simulink model "Systeem_Identificatie_Parameter_Estimation"  (R2018b)
settings: Solver=FixedStepAuto  StartTime=0.0  StopTime=4  FixedStep=1/50000  RelTol=1e-3
values from neighbouring files (symbols this model uses):
  bg = 18.2e-6    (= 1.82e-05)    [Data_conversion.m]
  bm = 18.2e-6    (= 1.82e-05)    [Data_conversion.m]
  Jg = 0.0000542    (= 5.42e-05)    [Data_conversion.m]
  Jm = 0.0000542    (= 5.42e-05)    [Data_conversion.m]
  Ke = (1/102)*(60/(2*pi))    (= 0.0936205547599)    [Data_conversion.m]
  Kt = 93.4e-3    (= 0.0934)    [Data_conversion.m]
  La = 0.423e-3    (= 0.000423)    [Data_conversion.m]
  n = 16.5    [Data_conversion.m]
  Ra = 0.608    [Data_conversion.m]
settings Model: Creator=BooJC  LastModifiedBy=Roberto
settings DataIOCC: ExternalInput=voltageTime  LoadExternalInput=on  DSMLogging=off
settings DebuggingCC: LibraryContextMissingDiagnostic=none
settings SFSimCC: SimUseLocalCustomCode=off
settings RTWCC: RTWUseLocalCustomCode=off

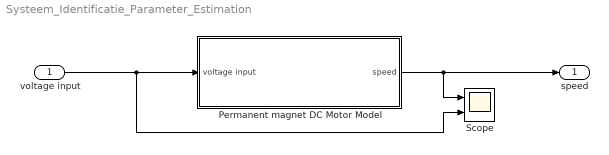
== system Systeem_Identificatie_Parameter_Estimation ==
  voltage input : Inport
  Permanent magnet DC Motor Model : Subsystem
  Scope : Scope  NumInputPorts=2
  speed : Outport
  wires:
  Permanent magnet DC Motor Model/1(speed) -> Scope/1, speed/1
  voltage input/1 -> Scope/2, Permanent magnet DC Motor Model/1(voltage input)

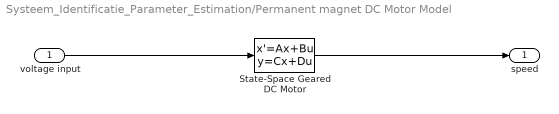
== system Systeem_Identificatie_Parameter_Estimation/Permanent magnet DC Motor Model ==
  voltage input : Inport
  State-Space Geared DC Motor : StateSpace  A=[-(bm*(n^2) + bg)/(Jm*(n^2) + Jg) Kt*n/(Jm*(n^2) + Jg); -(n*Ke)/La -Ra/La]  B=[0; 1/La]  C=[1 0]  D=0  InitialCondition=0  ContinuousStateAttributes='Speed'
  speed : Outport
  wires:
  State-Space Geared DC Motor/1 -> speed/1
  voltage input/1 -> State-Space Geared DC Motor/1
